simulink model "costas_pYll_BPSK"  (Simulink 8.4)
settings: Solver=VariableStepDiscrete  StartTime=0.0  StopTime=inf  RelTol=1e-3
libraries: dsparch4 x5, simulink x3, commchan3 x2, commsynccomp2 x2, dspsrcs4 x2, commrandsrc2 x1, commsink2 x1, commutil2 x1
settings Model: Creator=Lekha1  LastModifiedBy=Ben
settings OptimizationCC: InitFltsAndDblsToZero=on

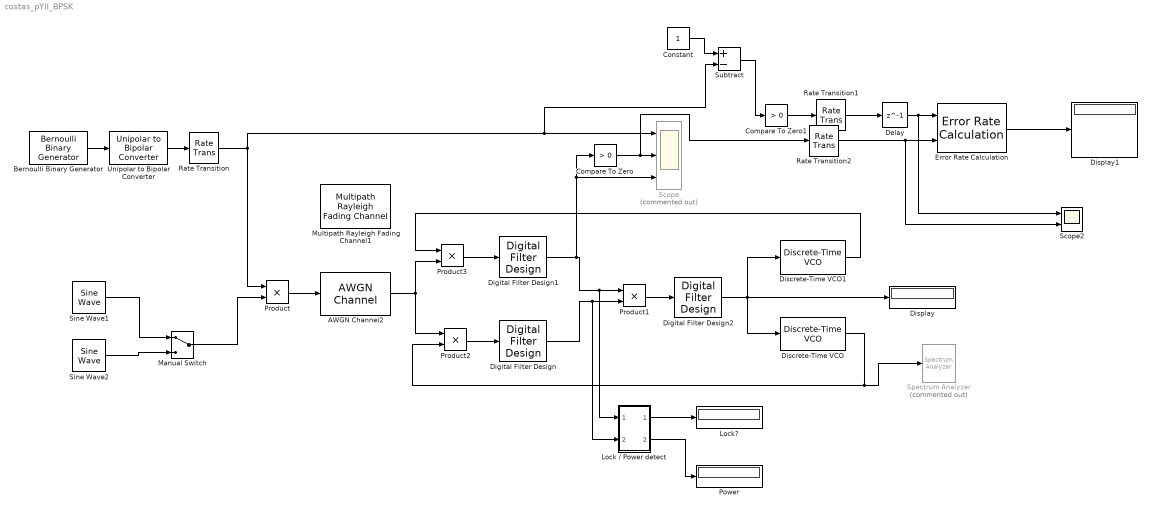
== system costas_pYll_BPSK ==
  AWGN Channel2 : commchan3/AWGN Channel  InputProcessing=Inherited (this choice will be removed - see release notes)  seed=67  noiseMode="Signal to noise ratio  (SNR)"  EbNodB=10  EsNodB=10  SNRdB=10  bitsPerSym=1  Ps=1  Tsym=1  variance=1
  Bernoulli Binary Generator : commrandsrc2/Bernoulli Binary Generator  P=0.5  seed=61  Ts=1/200  frameBased=off  sampPerFrame=1  orient=off  outDataType=double
  Compare To Zero : simulink/Logic and Bit Operations/Compare To Zero  relop=>  OutDataTypeStr=uint8  ZeroCross=off
  Compare To Zero1 : simulink/Logic and Bit Operations/Compare To Zero  relop=>  OutDataTypeStr=uint8  ZeroCross=off
  Constant : Constant
  Delay : Delay  DelayLength=1  InitialCondition=0
  Digital Filter Design : dsparch4/Digital Filter Design  mwdsp_browser_bugfix_var=off
  Digital Filter Design1 : dsparch4/Digital Filter Design  mwdsp_browser_bugfix_var=off
  Digital Filter Design2 : dsparch4/Digital Filter Design  mwdsp_browser_bugfix_var=off
  Discrete-Time VCO : commsynccomp2/Discrete-Time VCO  Ac=1  Fc=1e3  Kc=1e2  Ph=pi/2  ts=1/16e3
  Discrete-Time VCO1 : commsynccomp2/Discrete-Time VCO  Ac=1  Fc=1e3  Kc=1e2  Ph=0  ts=1/16e3
  Display : Display
  Display1 : Display
  Error Rate Calculation : commsink2/Error Rate Calculation  N=0  st_delay=1  cp_mode=Entire frame  subframe=[]  PMode=Port  WsName=QAM_BER  RsMode2=off  stop=off  numErr=maxerr  maxBits=maxbits
  Lock / Power detect : Subsystem
  Lock? : Display
  Manual Switch : ManualSwitch
  Multipath Rayleigh Fading Channel1 : commchan3/Multipath Rayleigh Fading Channel  maxDopplerShift=40  spectrumType=Jakes  sigmaGaussian=1/sqrt(2)  coeffRounded=[1 -1.72 0.785]  freqMinMaxRJakes=[0 1]  freqMinMaxAJakes=[0 1]  sigmaGaussian1=1/sqrt(2)  sigmaGaussian2=1/sqrt(2)  centerFreqGaussian1=0.0  centerFreqGaussian2=0.0  gainGaussian1=0.5  gainGaussian2=0.5  coeffBell=9  dopplerSpectrum=doppler.jakes  pathDelays=[0 2e-6]  avgPathGaindB=[0 -3]  normalizePathGains=on  seed=73  enableProbe=0  openVisAtStart=off  outPathGains=off  outDelay=off
  Power : Display
  Product{,1..3} (4 alike) : Product  RndMeth=Zero
  Rate Transition : RateTransition
  Rate Transition1 : RateTransition  OutPortSampleTime=1/200
  Rate Transition2 : RateTransition  OutPortSampleTime=1/200
  Scope : Scope  Commented=on  NumInputPorts=3
      settings: TimeRange=0.5  YMin=-1~0~-1  YMax=1~1~1
  Scope2 : Scope  NumInputPorts=2
      settings: TimeRange=0.5  YMin=0~0  YMax=1~1  SaveName=ScopeData2
  Sine Wave1 : dspsrcs4/Sine Wave  Amplitude=1  Frequency=2e3  Phase=0  SampleMode=Discrete  OutComplex=Real  CompMethod=Trigonometric fcn  TableSize=Speed  SampleTime=1/(16*2e3)  SamplesPerFrame=1  ResetState=Restart at time zero  dataType=double  wordLen=16  udDataType=sfix(16)  fracBitsMode=Best precision  numFracBits=15  OutDataTypeStr=double  LastOutDataTypeStr=double
  Sine Wave2 : dspsrcs4/Sine Wave  Amplitude=1  Frequency=2.1002e3  Phase=0  SampleMode=Discrete  OutComplex=Real  CompMethod=Trigonometric fcn  TableSize=Speed  SampleTime=1/(16*2e3)  SamplesPerFrame=1  ResetState=Restart at time zero  dataType=double  wordLen=16  udDataType=sfix(16)  fracBitsMode=Best precision  numFracBits=15  OutDataTypeStr=double  LastOutDataTypeStr=double
  Spectrum Analyzer : SpectrumAnalyzer  Commented=on
  Subtract : Sum  Inputs=+-
  Unipolar to Bipolar Converter : commutil2/Unipolar to Bipolar Converter  M=2  polarity=Positive  dataType=Same as input
  wires:
  Product/1 -> AWGN Channel2/1
  Digital Filter Design1/1 -> Lock / Power detect/1(In1), Product1/1, Scope/3, Compare To Zero/1
  Digital Filter Design/1 -> Lock / Power detect/2(In2), Product1/2
  Product1/1 -> Digital Filter Design2/1
  Digital Filter Design2/1 -> Display/1, Discrete-Time VCO1/1, Discrete-Time VCO/1
  Product2/1 -> Digital Filter Design/1
  Product3/1 -> Digital Filter Design1/1
  Discrete-Time VCO1/1 -> Product3/1
  Discrete-Time VCO/1 -> Product2/2, Spectrum Analyzer/1
  Rate Transition/1 -> Subtract/2, Scope/1, Product/1
  Bernoulli Binary Generator/1 -> Unipolar to Bipolar Converter/1
  Unipolar to Bipolar Converter/1 -> Rate Transition/1
  Compare To Zero/1 -> Rate Transition2/1, Scope/2
  AWGN Channel2/1 -> Product3/2, Product2/1
  Manual Switch/1 -> Product/2
  Sine Wave1/1 -> Manual Switch/1
  Sine Wave2/1 -> Manual Switch/2
  Error Rate Calculation/1 -> Display1/1
  Constant/1 -> Subtract/1
  Subtract/1 -> Compare To Zero1/1
  Compare To Zero1/1 -> Rate Transition1/1
  Rate Transition1/1 -> Delay/1
  Rate Transition2/1 -> Scope2/2, Error Rate Calculation/2
  Delay/1 -> Scope2/1, Error Rate Calculation/1
  Lock / Power detect/1(Out1) -> Lock?/1
  Lock / Power detect/2(Out2) -> Power/1

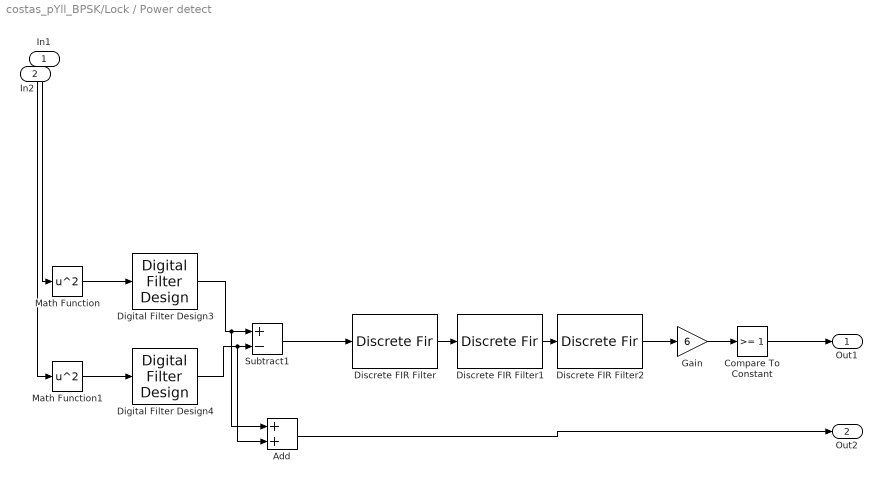
== system costas_pYll_BPSK/Lock / Power detect ==
  In1 : Inport
  In2 : Inport  Port=2
  Add : Sum
  Compare To Constant : simulink/Logic and Bit Operations/Compare To Constant  relop=>=  const=1  OutDataTypeStr=boolean
  Digital Filter Design3 : dsparch4/Digital Filter Design  mwdsp_browser_bugfix_var=off
  Digital Filter Design4 : dsparch4/Digital Filter Design  mwdsp_browser_bugfix_var=off
  Discrete FIR Filter : DiscreteFir  Coefficients=[0.01 0.01 0.01 0.01 0.01 0.01 0.01 0.01 0.01 0.01 0.01 0.01 0.01 0.01 0.01 0.01 0.01 0.01 0.01 0.01 0.01 0.01 0.01 0.01 0.01 0.01 0.01 0.01 0.01 0.01 0.01 0.01 0.01 0.01 0.01 0.01 0.01 0.01 0.01 0.01 0.01 0.01 0.01 0.01 0.01 0.01 0.01 0.01 0.01 0.01 0.01 0.01 0.01 0.01 0.01 0.01 0.01 0.01 0.01 0.01 0.01 0.01 0.01 0.01 0.01 0.01 0.01 0.01 0.01 0.01 0.01 0.01 0.01 0.01 0.01 0.01 0.01 0.01 0.01 0.01 0.01 0.01 0.01 0.01 0.01 0.01 0.01 0.01 0.01 0.01 0.01 0.01 0.01 0.01 0.01 0.01 0.01 0.01 0.01 0.01]  InputProcessing=Columns as channels (frame based)
  Discrete FIR Filter1 : DiscreteFir  Coefficients=[0.01 0.01 0.01 0.01 0.01 0.01 0.01 0.01 0.01 0.01 0.01 0.01 0.01 0.01 0.01 0.01 0.01 0.01 0.01 0.01 0.01 0.01 0.01 0.01 0.01 0.01 0.01 0.01 0.01 0.01 0.01 0.01 0.01 0.01 0.01 0.01 0.01 0.01 0.01 0.01 0.01 0.01 0.01 0.01 0.01 0.01 0.01 0.01 0.01 0.01 0.01 0.01 0.01 0.01 0.01 0.01 0.01 0.01 0.01 0.01 0.01 0.01 0.01 0.01 0.01 0.01 0.01 0.01 0.01 0.01 0.01 0.01 0.01 0.01 0.01 0.01 0.01 0.01 0.01 0.01 0.01 0.01 0.01 0.01 0.01 0.01 0.01 0.01 0.01 0.01 0.01 0.01 0.01 0.01 0.01 0.01 0.01 0.01 0.01 0.01]  InputProcessing=Columns as channels (frame based)
  Discrete FIR Filter2 : DiscreteFir  Coefficients=[0.01 0.01 0.01 0.01 0.01 0.01 0.01 0.01 0.01 0.01 0.01 0.01 0.01 0.01 0.01 0.01 0.01 0.01 0.01 0.01 0.01 0.01 0.01 0.01 0.01 0.01 0.01 0.01 0.01 0.01 0.01 0.01 0.01 0.01 0.01 0.01 0.01 0.01 0.01 0.01 0.01 0.01 0.01 0.01 0.01 0.01 0.01 0.01 0.01 0.01 0.01 0.01 0.01 0.01 0.01 0.01 0.01 0.01 0.01 0.01 0.01 0.01 0.01 0.01 0.01 0.01 0.01 0.01 0.01 0.01 0.01 0.01 0.01 0.01 0.01 0.01 0.01 0.01 0.01 0.01 0.01 0.01 0.01 0.01 0.01 0.01 0.01 0.01 0.01 0.01 0.01 0.01 0.01 0.01 0.01 0.01 0.01 0.01 0.01 0.01]  InputProcessing=Columns as channels (frame based)
  Gain : Gain  Gain=6
  Math Function : Math  Operator=square  SaturateOnIntegerOverflow=on
  Math Function1 : Math  Operator=square  SaturateOnIntegerOverflow=on
  Subtract1 : Sum  Inputs=+-
  Out1 : Outport
  Out2 : Outport  Port=2
  wires:
  Digital Filter Design4/1 -> Add/2, Subtract1/2
  Math Function/1 -> Digital Filter Design3/1
  Digital Filter Design3/1 -> Add/1, Subtract1/1
  Math Function1/1 -> Digital Filter Design4/1
  Discrete FIR Filter2/1 -> Gain/1
  Gain/1 -> Compare To Constant/1
  In1/1 -> Math Function/1
  Add/1 -> Out2/1
  Discrete FIR Filter1/1 -> Discrete FIR Filter2/1
  In2/1 -> Math Function1/1
  Subtract1/1 -> Discrete FIR Filter/1
  Compare To Constant/1 -> Out1/1
  Discrete FIR Filter/1 -> Discrete FIR Filter1/1
